simulink model "mymodel"  (R2020a)
settings: Solver=VariableStepAuto  StartTime=0.0  StopTime=10.0  RelTol=1e-3
values from neighbouring files (symbols this model uses):
  XIC = [U_init V_init W_init P_init Q_init R_init PHI_init THETA_init PSSI_init X_init     Y_init Z_init]'    [run_openloopsim_revisedinput.m]
settings Model: Creator=Farhat  LastModifiedBy=AbdulRahim
settings DataIOCC: ReturnWorkspaceOutputs=off
settings DebuggingCC: ArithmeticOperatorsInVariantConditions=warning
settings SFSimCC: SimUseLocalCustomCode=off  CustomCodeUndefinedFunction=UseInterfaceOnly
settings RTWCC: RTWUseLocalCustomCode=off
settings CodeAppCC: StateflowObjectComments=on

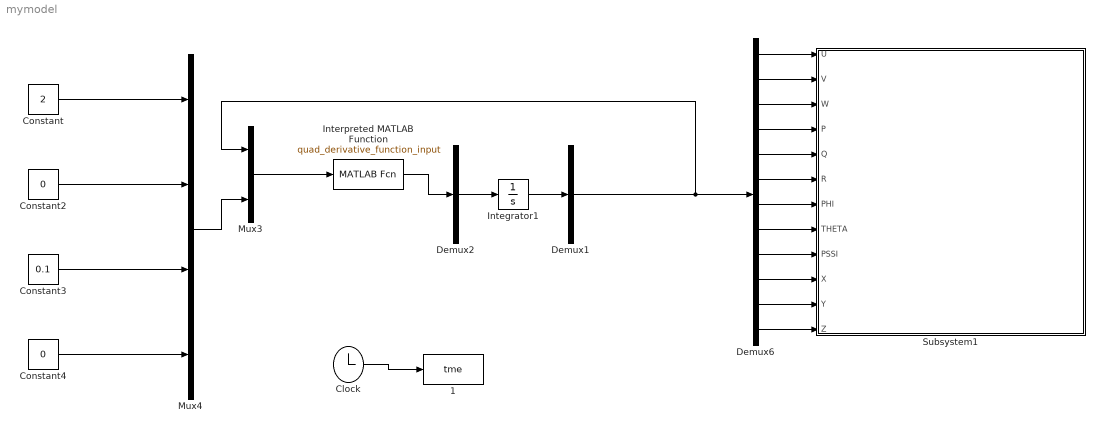
== system mymodel ==
  1 : ToWorkspace  VariableName=tme  SampleTime=-1
  Clock : Clock
  Constant : Constant  Value=2
  Constant2 : Constant  Value=0
  Constant3 : Constant  Value=0.1
  Constant4 : Constant  Value=0
  Demux1 : Demux  Outputs=[12 ]
  Demux2 : Demux  Outputs=[12]
  Demux6 : Demux  Outputs=[1 1 1 1 1 1 1 1 1 1 1 1]
  Integrator1 : Integrator  InitialCondition=XIC
  Interpreted MATLAB Function : MATLABFcn  MATLABFcn=quad_derivative_function_input  OutputDimensions=12
  Mux3 : Mux  Inputs=[12 4 ]
  Mux4 : Mux
  Subsystem1 : Subsystem
  wires:
  Integrator1/1 -> Demux1/1
  Mux4/1 -> Mux3/2
  Mux3/1 -> Interpreted MATLAB Function/1
  Interpreted MATLAB Function/1 -> Demux2/1
  Demux2/1 -> Integrator1/1
  Constant4/1 -> Mux4/4
  Constant2/1 -> Mux4/2
  Constant/1 -> Mux4/1
  Constant3/1 -> Mux4/3
  Demux6/1 -> Subsystem1/1(U)
  Demux6/2 -> Subsystem1/2(V)
  Demux6/3 -> Subsystem1/3(W)
  Demux6/4 -> Subsystem1/4("P ")
  Demux6/5 -> Subsystem1/5("Q ")
  Demux6/6 -> Subsystem1/6(R)
  Demux6/7 -> Subsystem1/7(PHI)
  Demux6/8 -> Subsystem1/8(THETA)
  Demux6/9 -> Subsystem1/9(PSSI)
  Demux6/10 -> Subsystem1/10(X)
  Demux6/11 -> Subsystem1/11(Y)
  Demux6/12 -> Subsystem1/12(Z)
  Demux1/1 -> Mux3/1, Demux6/1
  Clock/1 -> 1/1

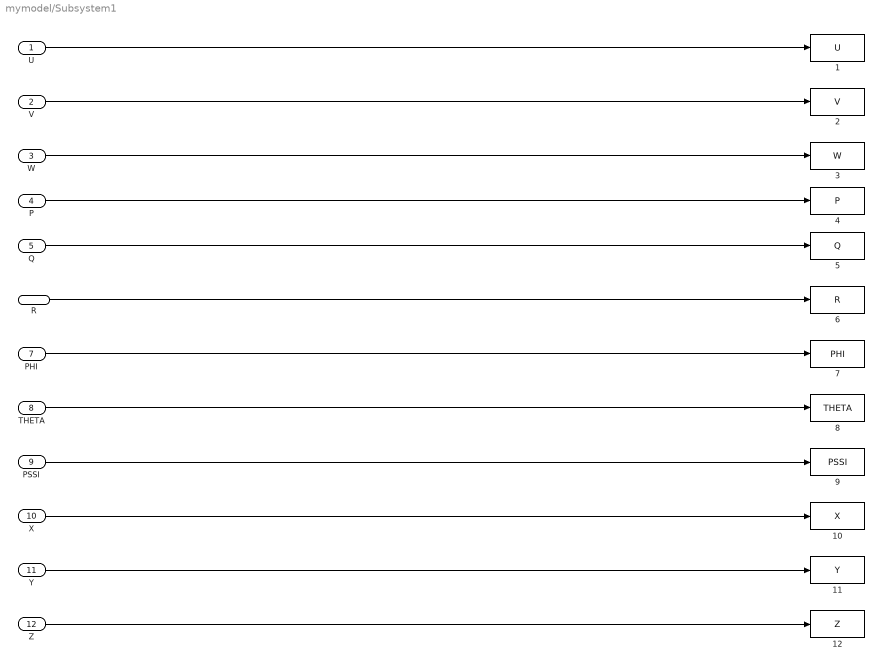
== system mymodel/Subsystem1 ==
  U : Inport
  V : Inport  Port=2
  W : Inport  Port=3
  "P " : Inport  Port=4
  "Q " : Inport  Port=5
  R : Inport  Port=6
  PHI : Inport  Port=7
  THETA : Inport  Port=8
  PSSI : Inport  Port=9
  X : Inport  Port=10
  Y : Inport  Port=11
  Z : Inport  Port=12
  1 : ToWorkspace  VariableName=U  SampleTime=-1
  10 : ToWorkspace  VariableName=X  SampleTime=-1
  11 : ToWorkspace  VariableName=Y  SampleTime=-1
  "12 " : ToWorkspace  VariableName=Z  SampleTime=-1
  2 : ToWorkspace  VariableName=V  SampleTime=-1
  3 : ToWorkspace  VariableName=W  SampleTime=-1
  4 : ToWorkspace  VariableName=P  SampleTime=-1
  5 : ToWorkspace  VariableName=Q  SampleTime=-1
  6 : ToWorkspace  VariableName=R  SampleTime=-1
  7 : ToWorkspace  VariableName=PHI  SampleTime=-1
  8 : ToWorkspace  VariableName=THETA  SampleTime=-1
  9 : ToWorkspace  VariableName=PSSI  SampleTime=-1
  wires:
  Z/1 -> "12 "/1
  "Q "/1 -> 5/1
  Y/1 -> 11/1
  U/1 -> 1/1
  THETA/1 -> 8/1
  X/1 -> 10/1
  V/1 -> 2/1
  R/1 -> 6/1
  PHI/1 -> 7/1
  PSSI/1 -> 9/1
  W/1 -> 3/1
  "P "/1 -> 4/1
